simulink model "understandingof_tangentwave"  (R2024b)
settings: Solver=VariableStepAuto  StartTime=0.0  StopTime=10.0  MaxStep=0.01  RelTol=1e-3
settings Model: Creator=admin  LastModifiedBy=admin

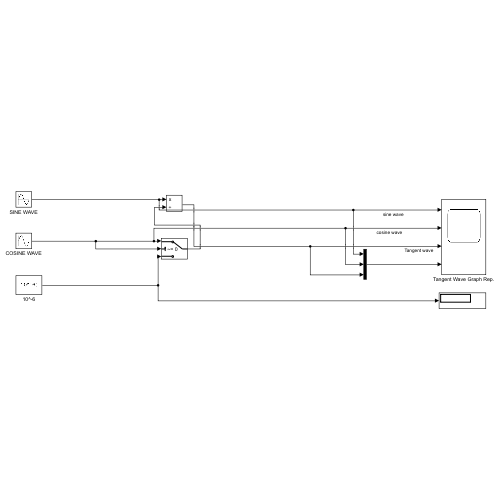
[thumbnail: Simulink's stored preview of the top-level diagram]
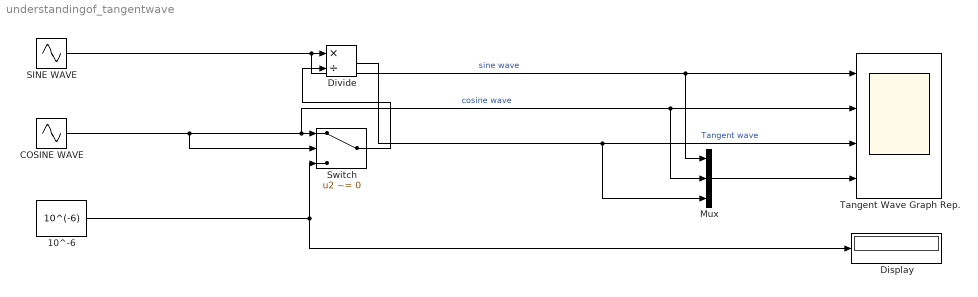
== system understandingof_tangentwave ==
  10^-6 : Constant  Value=10^(-6)
  COSINE WAVE : Sin  Phase=pi/2  SampleTime=0
  Display : Display
  Divide : Product  Inputs=*/
  Mux : Mux  Inputs=3
  SINE WAVE : Sin  SampleTime=0
  Switch : Switch  Criteria=u2 ~= 0  SaturateOnIntegerOverflow=off  InputSameDT=off
  Tangent Wave Graph Rep. : Scope  NumInputPorts=4
  wires:
  SINE WAVE/1 -> Mux/1, Tangent Wave Graph Rep./1, Divide/1  "sine wave"
  Divide/1 -> Tangent Wave Graph Rep./3, Mux/3  "Tangent wave"
  COSINE WAVE/1 -> Switch/2, Mux/2, Tangent Wave Graph Rep./2, Switch/1  "cosine wave"
  10^-6/1 -> Display/1, Switch/3
  Switch/1 -> Divide/2
  Mux/1 -> Tangent Wave Graph Rep./4
